simulink model "systolic_8_tap"  (R2021a)
settings: Solver=VariableStepAuto  StartTime=0.0  StopTime=4000  RelTol=1e-3
undefined symbols (not defined in the file): variable_step_size_calc, x1
libraries: dspsrcs4 x4, dspstat3 x4, dspmathops x2
settings Model: Creator=HP  LastModifiedBy=HP

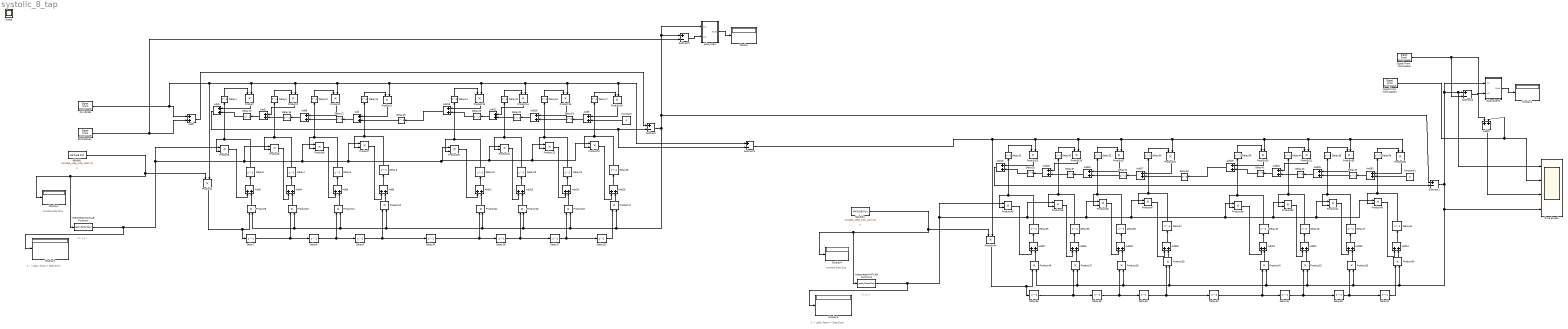
== system systolic_8_tap ==
  note: Variable Step Size
  note: μ
  note: ( 1- μ γ )
  note: 1 - ( Leaky factor * Step Size )
  note: Variable Step Size
  note: μ
  note: ( 1- μ γ )
  note: 1 - ( Leaky factor * Step Size )
  Add{,1..33} (34 alike) : Sum
  Constant : Constant  Value=0
  Constant1 : Constant  Value=0
  Delay{1..60} (60 alike) : Delay  DelayLength=1  InitialCondition=0
  Display{,1..5} (6 alike) : Display
      Display3 settings: Format=decimal (Stored Integer)
      Display5 settings: Format=decimal (Stored Integer)
  ECG SIGNAL : dspsrcs4/Signal From Workspace  X=m1  Ts=1  nsamps=1  OutputAfterFinalValue=Setting to zero  ignoreOrWarnInputAndFrameLengths=off  OutputFrames=off
  Interpreted MATLAB Function : MATLABFcn  MATLABFcn=LeakyFactorCalc
  Interpreted MATLAB Function1 : MATLABFcn  MATLABFcn=LeakyFactorCalc
  PLI NOISE : dspsrcs4/Signal From Workspace  X=x1  Ts=1  nsamps=1  OutputAfterFinalValue=Setting to zero  ignoreOrWarnInputAndFrameLengths=off  OutputFrames=off
  Product{,1..49} (50 alike) : Product
  Signal From Workspace : dspsrcs4/Signal From Workspace  X=m1  Ts=1  nsamps=1  OutputAfterFinalValue=Setting to zero  ignoreOrWarnInputAndFrameLengths=off  OutputFrames=off
  Signal From Workspace1 : dspsrcs4/Signal From Workspace  X=x1  Ts=1  nsamps=1  OutputAfterFinalValue=Setting to zero  ignoreOrWarnInputAndFrameLengths=off  OutputFrames=off
  Subsystem : Subsystem
  Subsystem1 : Subsystem
  Subtract{,1..4} (5 alike) : Sum  Inputs=+-
  Time Scope1 : Scope  NumInputPorts=4
  fdlkjfkfj : MATLABFcn  MATLABFcn=variable_step_size_calc(x1)
  fdlkjfkfj1 : MATLABFcn  MATLABFcn=variable_step_size_calc(x1)
  Scope : Scope
  wires:
  Product6/1 -> Add4/1
  Product9/1 -> Add3/2
  Product5/1 -> Add3/1
  Product4/1 -> Product9/1, Delay7/1
  Delay9/1 -> Delay30/1, Product12/1
  Product12/1 -> Add6/2
  Product8/1 -> Add5/1
  Delay5/1 -> Product8/2, Delay10/1
  Product7/1 -> Add6/1
  Product10/1 -> Add4/2
  Subsystem/1(Out1) -> Display/1
  Delay7/1 -> Product10/1, Delay8/1
  Delay6/1 -> Product7/2, Delay11/1
  ECG SIGNAL/1 -> Add7/2, Subtract2/2
  Delay4/1 -> Delay2/1, Product6/2
  Subtract2/1 -> Subsystem/2(In2)
  Add6/1 -> Delay6/1
  Delay8/1 -> Product11/1, Delay9/1
  fdlkjfkfj/1 -> Product4/1, Interpreted MATLAB Function/1, Display2/1
  Add3/1 -> Delay3/1
  Interpreted MATLAB Function/1 -> Display3/1, Product5/1, Product6/1, Product8/1, Product7/1, Product21/1, Product23/1, Product22/1, Product20/1
  Add4/1 -> Delay4/1
  Product11/1 -> Add5/2
  Add5/1 -> Delay5/1
  Delay3/1 -> Delay1/1, Product5/2
  Delay2/1 -> Product1/1
  Delay10/1 -> Product2/1
  Delay11/1 -> Product3/1
  Delay1/1 -> Product/1
  Delay29/1 -> Add/2
  Product3/1 -> Add/1
  Add/1 -> Delay12/1
  Delay12/1 -> Add8/2
  Product2/1 -> Add8/1
  Add8/1 -> Delay15/1
  Delay15/1 -> Add2/2
  Product1/1 -> Add2/1
  Add2/1 -> Delay13/1
  Delay13/1 -> Add1/2
  Product/1 -> Add1/1
  Add14/1 -> Delay24/1
  Add13/1 -> Delay23/1
  Product13/1 -> Add10/1
  Delay19/1 -> Add10/2
  Product19/1 -> Add9/1
  Delay22/1 -> Delay14/1, Product20/2
  Delay20/1 -> Add11/2
  Delay24/1 -> Product23/2, Delay16/1
  Product18/1 -> Add16/1
  Delay25/1 -> Product22/2, Delay17/1
  Product20/1 -> Add12/1
  Constant/1 -> Add9/2
  Add11/1 -> Delay19/1
  Delay18/1 -> Add16/2
  Delay17/1 -> Product19/1
  Delay14/1 -> Product13/1
  Product16/1 -> Add14/2
  Add15/1 -> Delay25/1
  Product21/1 -> Add13/1
  Add12/1 -> Delay22/1
  Product17/1 -> Add15/2
  Delay21/1 -> Product14/1
  Product15/1 -> Add13/2
  Product22/1 -> Add15/1
  Delay23/1 -> Delay21/1, Product21/2
  Delay28/1 -> Product17/1
  Add9/1 -> Delay18/1
  Product14/1 -> Add11/1
  Product23/1 -> Add14/1
  Add16/1 -> Delay20/1
  Product24/1 -> Add12/2
  Delay16/1 -> Product18/1
  PLI NOISE/1 -> Add7/1, Subtract4/1, Product19/2, Product18/2, Product14/2, Product13/2, Product3/2, Product2/2, Product1/2, Product/2, Product4/2
  Add10/1 -> Delay29/1
  Delay30/1 -> Product24/1, Delay26/1
  Add1/1 -> Subtract4/2, Subtract/2
  Add7/1 -> Subtract/1
  Delay26/1 -> Product15/1, Delay27/1
  Delay27/1 -> Product16/1, Delay28/1
  Product29/1 -> Add30/2
  Delay41/1 -> Add19/2
  Interpreted MATLAB Function1/1 -> Display5/1, Product45/1, Product46/1, Product48/1, Product47/1, Product39/1, Product41/1, Product40/1, Product38/1
  Add29/1 -> Delay56/1
  Product31/1 -> Add20/1
  Add27/1 -> Delay53/1
  Add24/1 -> Delay48/1
  fdlkjfkfj1/1 -> Product44/1, Interpreted MATLAB Function1/1, Display4/1
  Delay43/1 -> Add20/2
  Delay37/1 -> Add26/2
  Product42/1 -> Add21/2
  Delay54/1 -> Product42/1, Delay49/1
  Add32/1 -> Delay37/1
  Delay49/1 -> Product32/1, Delay50/1
  Delay39/1 -> Product36/1
  Delay56/1 -> Product48/2, Delay32/1
  Add20/1 -> Delay41/1
  Subtract/1 -> Subtract1/1, Subsystem/1(In1), Subtract2/1, Product17/2, Product16/2, Product15/2, Product24/2, Product12/2, Product11/2, Product10/2, Product9/2
  Add18/1 -> Subtract1/2
  Add21/1 -> Delay45/1
  Add19/1 -> Delay52/1
  Subtract4/1 -> Product36/2, Product35/2, Product31/2, Product30/2, Product43/2, Product37/2, Product26/2, Product25/2, Product44/2
  Delay38/1 -> Product35/1
  Subtract1/1 -> Subsystem1/1(In1), Time Scope1/1, Subtract3/1, Product34/2, Product33/2, Product32/2, Product42/2, Product29/2, Product28/2, Product27/2, Product49/2, Time Scope1/4
  Delay33/1 -> Product43/1
  Delay45/1 -> Delay36/1, Product38/2
  Delay60/1 -> Delay54/1, Product29/1
  Add26/1 -> Delay35/1
  Product43/1 -> Add17/1
  Add33/1 -> Delay40/1
  Delay51/1 -> Product34/1
  Product39/1 -> Add22/1
  Delay46/1 -> Delay44/1, Product39/2
  Add25/1 -> Delay43/1
  Delay53/1 -> Delay31/1, Product45/2
  Product41/1 -> Add23/1
  Delay47/1 -> Product41/2, Delay38/1
  Delay52/1 -> Add17/2
  Add17/1 -> Delay34/1
  Add30/1 -> Delay57/1
  Product36/1 -> Add33/1
  Product34/1 -> Add24/2
  Product45/1 -> Add27/1
  Product40/1 -> Add24/1
  Product25/1 -> Add18/1
  Product37/1 -> Add32/1
  Delay32/1 -> Product37/1
  Delay42/1 -> Product26/1
  Delay35/1 -> Add18/2
  Delay31/1 -> Product25/1
  Add28/1 -> Delay55/1
  Delay59/1 -> Product28/1, Delay60/1
  Subtract3/1 -> Subsystem1/2(In2)
  Delay36/1 -> Product30/1
  Product48/1 -> Add29/1
  Delay34/1 -> Add32/2
  Subsystem1/1(Out1) -> Display1/1
  Delay57/1 -> Product47/2, Delay33/1
  Product30/1 -> Add19/1
  Product28/1 -> Add29/2
  Product47/1 -> Add30/1
  Product44/1 -> Product49/1, Delay58/1
  Delay50/1 -> Product33/1, Delay51/1
  Delay55/1 -> Delay42/1, Product46/2
  Delay44/1 -> Product31/1
  Add22/1 -> Delay46/1
  Product26/1 -> Add26/1
  Product38/1 -> Add21/1
  Product49/1 -> Add27/2
  Product33/1 -> Add23/2
  Delay58/1 -> Product27/1, Delay59/1
  Product32/1 -> Add22/2
  Product27/1 -> Add28/2
  Delay40/1 -> Add25/2
  Product35/1 -> Add25/1
  Add23/1 -> Delay47/1
  Delay48/1 -> Product40/2, Delay39/1
  Product46/1 -> Add28/1
  Constant1/1 -> Add33/2
  Signal From Workspace/1 -> Add31/1, Subtract3/2
  Signal From Workspace1/1 -> Add31/2, Time Scope1/2
  Add31/1 -> Time Scope1/3

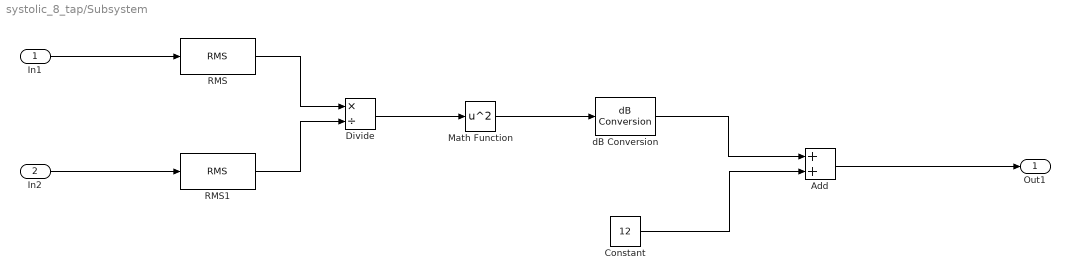
== system systolic_8_tap/Subsystem ==
  In1 : Inport
  In2 : Inport  Port=2
  Add : Sum
  Constant : Constant  Value=12
  Divide : Product  Inputs=*/
  Math Function : Math  Operator=square  SignedPower=on  OutputSignalType=real  SaturateOnIntegerOverflow=on
  RMS : dspstat3/RMS  run=on  directionMode=Each column  dimension=1  InputProcessing=Columns as channels (frame based)  reset_popup=None
  RMS1 : dspstat3/RMS  run=on  directionMode=Each column  dimension=1  InputProcessing=Columns as channels (frame based)  reset_popup=None
  dB Conversion : dspmathops/dB Conversion  dBtype=dB  intype=Amplitude  R=1  fuzz=off
  Out1 : Outport
  wires:
  RMS1/1 -> Divide/2
  dB Conversion/1 -> Add/1
  In1/1 -> RMS/1
  Divide/1 -> Math Function/1
  RMS/1 -> Divide/1
  In2/1 -> RMS1/1
  Add/1 -> Out1/1
  Constant/1 -> Add/2
  Math Function/1 -> dB Conversion/1

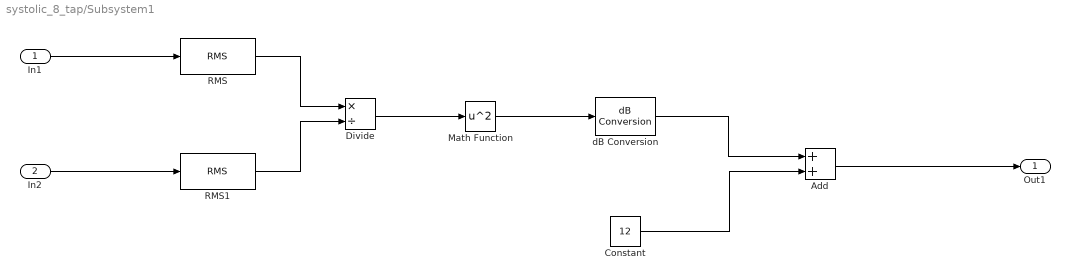
== system systolic_8_tap/Subsystem1 ==
  In1 : Inport
  In2 : Inport  Port=2
  Add : Sum
  Constant : Constant  Value=12
  Divide : Product  Inputs=*/
  Math Function : Math  Operator=square  SignedPower=on  OutputSignalType=real  SaturateOnIntegerOverflow=on
  RMS : dspstat3/RMS  run=on  directionMode=Each column  dimension=1  InputProcessing=Columns as channels (frame based)  reset_popup=None
  RMS1 : dspstat3/RMS  run=on  directionMode=Each column  dimension=1  InputProcessing=Columns as channels (frame based)  reset_popup=None
  dB Conversion : dspmathops/dB Conversion  dBtype=dB  intype=Amplitude  R=1  fuzz=off
  Out1 : Outport
  wires:
  RMS1/1 -> Divide/2
  dB Conversion/1 -> Add/1
  In1/1 -> RMS/1
  Divide/1 -> Math Function/1
  RMS/1 -> Divide/1
  In2/1 -> RMS1/1
  Add/1 -> Out1/1
  Constant/1 -> Add/2
  Math Function/1 -> dB Conversion/1
